simulink model "top_level_architecture"  (Simulink 8.5)
settings: Solver=ode45  StartTime=0.0  StopTime=10.0  RelTol=1e-3
settings Model: Creator=oezqk7  LastModifiedBy=tghx1e
settings DebuggingCC: SolverPrmCheckMsg=warning  FcnCallInpInsideContextMsg=UseLocalSettings

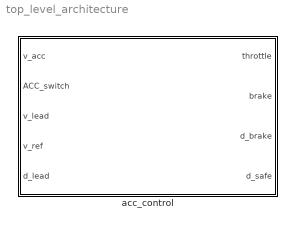
== system top_level_architecture ==
  acc_control : Subsystem

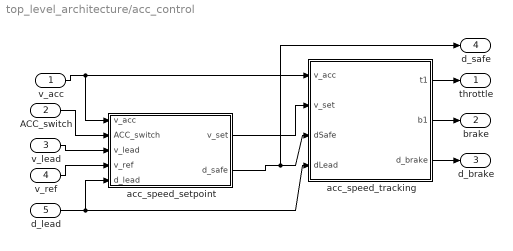
== system top_level_architecture/acc_control ==
  v_acc : Inport
  ACC_switch : Inport  Port=2
  v_lead : Inport  Port=3
  v_ref : Inport  Port=4
  d_lead : Inport  Port=5
  acc_speed_setpoint : Subsystem
  acc_speed_tracking : Subsystem
  throttle : Outport
  brake : Outport  Port=2
  d_brake : Outport  Port=3
  d_safe : Outport  Port=4
  wires:
  acc_speed_setpoint/1(v_set) -> acc_speed_tracking/2(v_set)
  acc_speed_tracking/1(t1) -> throttle/1
  v_lead/1 -> acc_speed_setpoint/3(v_lead)
  v_ref/1 -> acc_speed_setpoint/4(v_ref)
  acc_speed_tracking/2(b1) -> brake/1
  acc_speed_tracking/3(d_brake) -> d_brake/1
  d_lead/1 -> acc_speed_setpoint/5(d_lead), acc_speed_tracking/4(dLead)
  ACC_switch/1 -> acc_speed_setpoint/2(ACC_switch)
  v_acc/1 -> acc_speed_setpoint/1(v_acc), acc_speed_tracking/1(v_acc)
  acc_speed_setpoint/2(d_safe) -> acc_speed_tracking/3(dSafe), d_safe/1

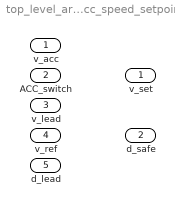
== system top_level_architecture/acc_control/acc_speed_setpoint ==
  v_acc : Inport
  ACC_switch : Inport  Port=2
  v_lead : Inport  Port=3
  v_ref : Inport  Port=4
  d_lead : Inport  Port=5
  v_set : Outport
  d_safe : Outport  Port=2

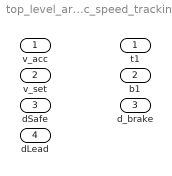
== system top_level_architecture/acc_control/acc_speed_tracking ==
  v_acc : Inport
  v_set : Inport  Port=2
  dSafe : Inport  Port=3
  dLead : Inport  Port=4
  t1 : Outport
  b1 : Outport  Port=2
  d_brake : Outport  Port=3
